simulink model "ODU_zad4"  (Simulink 6.3)
settings: Solver=ode45  StartTime=0.0  StopTime=4  RelTol=1e-3
settings Model: LastModifiedBy=Ms1

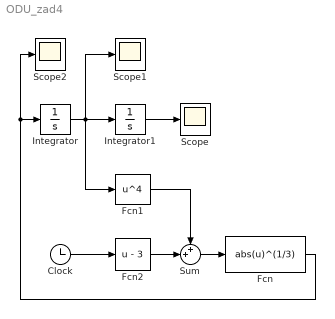
== system ODU_zad4 ==
  Clock : Clock
      settings: Decimation=10
  Fcn : Fcn  Expr=abs(u)^(1/3)
  Fcn1 : Fcn  Expr=u^4
  Fcn2 : Fcn  Expr=u - 3
  Integrator : Integrator  InitialCondition=-4
  Integrator1 : Integrator  InitialCondition=-5
  Scope : Scope
  Scope1 : Scope
  Scope2 : Scope
      settings: SaveName=ScopeData2
  Sum : Sum  Inputs=++|  SaturateOnIntegerOverflow=on  InputSameDT=on
  wires:
  Integrator/1 -> Integrator1/1, Fcn1/1, Scope1/1
  Integrator1/1 -> Scope/1
  Clock/1 -> Fcn2/1
  Sum/1 -> Fcn/1
  Fcn2/1 -> Sum/2
  Fcn1/1 -> Sum/1
  Fcn/1 -> Integrator/1, Scope2/1
